simulink model "blockdiag"  (R2018b)
settings: Solver=ode45  StartTime=0.0  StopTime=10.0  RelTol=1e-3  AbsTol=1e-6
undefined symbols (not defined in the file): C, L, R
settings Model: ExtModeTrigMode=oneshot  ExtModeArmWhenConnect=off  Creator=eechris  LastModifiedBy=eechris
settings DataIOCC: SaveFormat=Array  SignalLoggingSaveFormat=ModelDataLogs
settings OptimizationCC: BlockReduction=off  BooleanDataType=off
settings DebuggingCC: SaveWithParameterizedLinksMsg=none  UnderspecifiedInitializationDetection=Classic  MergeDetectMultiDrivingBlocksExec=none  SignalResolutionControl=TryResolveAllWithWarning  MultiTaskDSMMsg=warning  MultiTaskCondExecSysMsg=none
settings HardwareCC: TargetUnknown=on
settings ModelReferenceCC: PropagateSignalLabelsOutOfModel=off
settings GRTTargetCC: CombineOutputUpdateFcns=off  GRTInterface=on

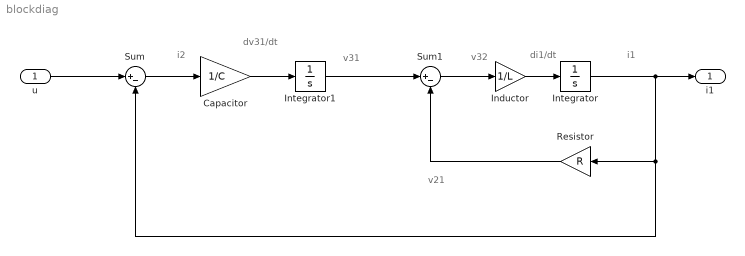
== system blockdiag ==
  note: dv31/dt
  note: v31
  note: v32
  note: di1/dt
  note: i1
  note: v21
  note: i2
  u : Inport
  Capacitor : Gain  Gain=1/C  OutDataTypeStr=Inherit: Same as input  ParamDataTypeStr=Inherit: Same as input
  Inductor : Gain  Gain=1/L  SaturateOnIntegerOverflow=on  OutDataTypeStr=Inherit: Same as input  ParamDataTypeStr=Inherit: Same as input
  Integrator : Integrator
  Integrator1 : Integrator
  Resistor : Gain  Gain=R  SaturateOnIntegerOverflow=on  OutDataTypeStr=Inherit: Same as input  ParamDataTypeStr=Inherit: Same as input
  Sum : Sum  Inputs=|+-  InputSameDT=on  OutDataTypeStr=Inherit: Same as first input
  Sum1 : Sum  Inputs=|+-  InputSameDT=on  OutDataTypeStr=Inherit: Same as first input
  i1 : Outport
  wires:
  Inductor/1 -> Integrator/1
  Sum1/1 -> Inductor/1
  Capacitor/1 -> Integrator1/1
  Sum/1 -> Capacitor/1
  Integrator/1 -> Resistor/1, Sum/2, i1/1
  u/1 -> Sum/1
  Integrator1/1 -> Sum1/1
  Resistor/1 -> Sum1/2
